simulink library "CTRL_UP_YAWACC"  (R2023b)
settings: Solver=VariableStepAuto  StartTime=0.0  StopTime=10.0  RelTol=1e-3
undefined symbols (not defined in the file): p_JzVeh_kgm2
settings Model: Creator=blatak  LastModifiedBy=blatak

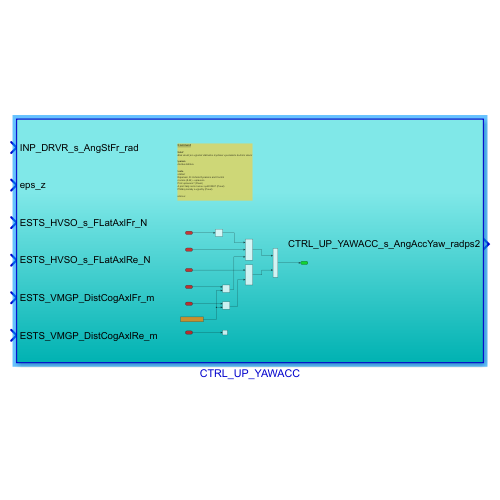
[thumbnail: Simulink's stored preview of the top-level diagram]
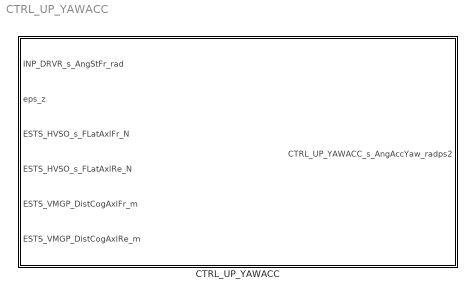
== system CTRL_UP_YAWACC ==
  CTRL_UP_YAWACC : Subsystem

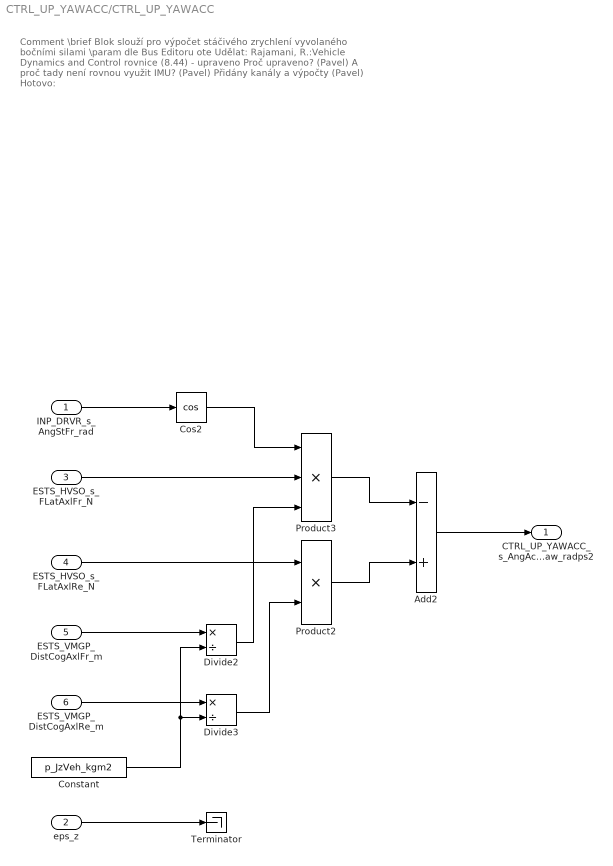
== system CTRL_UP_YAWACC/CTRL_UP_YAWACC ==
  note: Comment
      |
      | \brief
      | Blok slouží pro výpočet stáčivého zrychlení vyvolaného bočními silami
      |
      | \param
      | dle Bus Editoru
      |
      | \note
      | Udělat:
      | Rajamani, R.:Vehicle Dynamics and Control
      | rovnice (8.44) - upraveno
      | Proč upraveno? (Pavel)
      | A proč tady není rovnou využit IMU? (Pavel)
      | Přidány kanály a výpočty (Pavel)
      |
      | Hotovo:
  INP_DRVR_s_AngStFr_rad : Inport
  eps_z : Inport  Port=2
  ESTS_HVSO_s_FLatAxlFr_N : Inport  Port=3
  ESTS_HVSO_s_FLatAxlRe_N : Inport  Port=4
  ESTS_VMGP_DistCogAxlFr_m : Inport  Port=5
  ESTS_VMGP_DistCogAxlRe_m : Inport  Port=6
  Add2 : Sum  Inputs=-+
  Constant : Constant  Value=p_JzVeh_kgm2
  Cos2 : Trigonometry  Operator=cos
  Divide2 : Product  Inputs=*/
  Divide3 : Product  Inputs=*/
  Product2 : Product
  Product3 : Product  Inputs=3
  Terminator : Terminator
  CTRL_UP_YAWACC_s_AngAccYaw_radps2 : Outport
  wires:
  Divide2/1 -> Product3/3
  Product3/1 -> Add2/1
  ESTS_VMGP_DistCogAxlFr_m/1 -> Divide2/1
  ESTS_VMGP_DistCogAxlRe_m/1 -> Divide3/1
  ESTS_HVSO_s_FLatAxlRe_N/1 -> Product2/1
  INP_DRVR_s_AngStFr_rad/1 -> Cos2/1
  Add2/1 -> CTRL_UP_YAWACC_s_AngAccYaw_radps2/1
  Divide3/1 -> Product2/2
  Cos2/1 -> Product3/1
  Product2/1 -> Add2/2
  eps_z/1 -> Terminator/1
  Constant/1 -> Divide3/2, Divide2/2
  ESTS_HVSO_s_FLatAxlFr_N/1 -> Product3/2
